simulink model "quadrotorsmodel2_wrapper"  (R2024b)
settings: Solver=FixedStepAuto  StartTime=0.0  StopTime=SimulationTime  FixedStep=timestep  RelTol=1e-3
Description:
  | Temporary wrapper for PIL simulation
settings Model: Creator=supaw  LastModifiedBy=supaw
settings DataIOCC: ExternalInput=inputStructure  LoadExternalInput=on

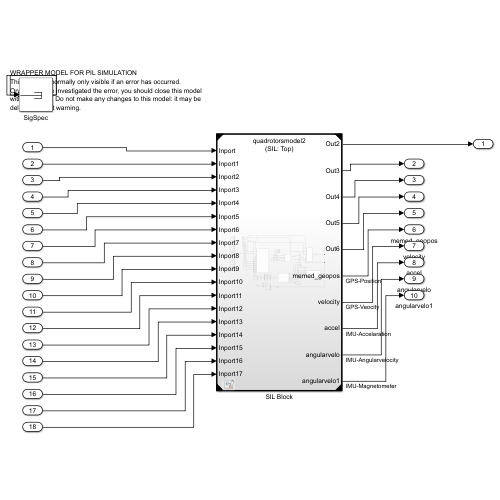
[thumbnail: Simulink's stored preview of the top-level diagram]
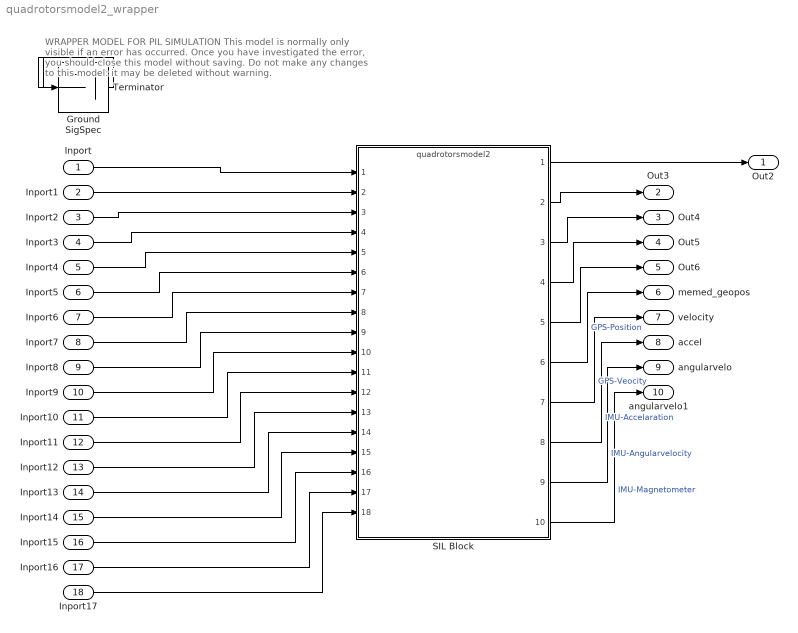
== system quadrotorsmodel2_wrapper ==
  note: WRAPPER MODEL FOR PIL SIMULATION
      | This model is normally only visible if an error has occurred.
      | Once you have investigated the error, you should close this model
      | without saving. Do not make any changes to this model: it may be
      | deleted without warning.
  Inport : Inport
  Inport1 : Inport  Port=2
  Inport2 : Inport  Port=3
  Inport3 : Inport  Port=4
  Inport4 : Inport  Port=5
  Inport5 : Inport  Port=6
  Inport6 : Inport  Port=7
  Inport7 : Inport  Port=8
  Inport8 : Inport  Port=9
  Inport9 : Inport  Port=10
  Inport10 : Inport  Port=11
  Inport11 : Inport  Port=12
  Inport12 : Inport  Port=13
  Inport13 : Inport  Port=14
  Inport14 : Inport  Port=15
  Inport15 : Inport  Port=16
  Inport16 : Inport  Port=17
  Inport17 : Inport  Port=18
  Ground : Ground
  SIL Block : ModelReference  ModelNameDialog=quadrotorsmodel2  SimulationMode=Software-in-the-loop (SIL)  CodeInterface=Top model  ModelReferenceVersion=1.2
  SigSpec : SignalSpecification  OutDataTypeStr=int32  Dimensions=1
  Terminator : Terminator
  Out2 : Outport
  Out3 : Outport  Port=2
  Out4 : Outport  Port=3
  Out5 : Outport  Port=4
  Out6 : Outport  Port=5
  memed_geopos : Outport  Port=6
  velocity : Outport  Port=7
  accel : Outport  Port=8
  angularvelo : Outport  Port=9
  angularvelo1 : Outport  Port=10
  wires:
  Inport/1 -> SIL Block/1
  Inport1/1 -> SIL Block/2
  Inport2/1 -> SIL Block/3
  Inport3/1 -> SIL Block/4
  Inport4/1 -> SIL Block/5
  Inport5/1 -> SIL Block/6
  Inport6/1 -> SIL Block/7
  Inport7/1 -> SIL Block/8
  Inport8/1 -> SIL Block/9
  Inport9/1 -> SIL Block/10
  Inport10/1 -> SIL Block/11
  Inport11/1 -> SIL Block/12
  Inport12/1 -> SIL Block/13
  Inport13/1 -> SIL Block/14
  Inport14/1 -> SIL Block/15
  Inport15/1 -> SIL Block/16
  Inport16/1 -> SIL Block/17
  Inport17/1 -> SIL Block/18
  SIL Block/1 -> Out2/1
  SIL Block/2 -> Out3/1
  SIL Block/3 -> Out4/1
  SIL Block/4 -> Out5/1
  SIL Block/5 -> Out6/1
  SIL Block/6 -> memed_geopos/1  "GPS-Position"
  SIL Block/7 -> velocity/1  "GPS-Veocity"
  SIL Block/8 -> accel/1  "IMU-Accelaration"
  SIL Block/9 -> angularvelo/1  "IMU-Angularvelocity"
  SIL Block/10 -> angularvelo1/1  "IMU-Magnetometer"
  Ground/1 -> SigSpec/1
  SigSpec/1 -> Terminator/1
